simulink model "EEE4022S_Double_Pendulum_Swing_Up_SIM"  (R2021a)
settings: Solver=ode4  StartTime=0.0  StopTime=10  FixedStep=0.002  RelTol=1e-3
values from neighbouring files (symbols this model uses):
  g = 9.81    [EEE4022S_Double_Inverted_Pendulum_Model.m]    (also in MediumPenModelling.m; ShortPenModelling.m)
  K = lqr(A,B,Q,R)    [EEE4022S_Double_Inverted_Pendulum_Model.m]
  L1 = 0.2096    [EEE4022S_Double_Inverted_Pendulum_Model.m]
  l1 = 0.1483    [EEE4022S_Double_Inverted_Pendulum_Model.m]
  l2 = 0.1778    [EEE4022S_Double_Inverted_Pendulum_Model.m]
  m1 = 0.25244    [EEE4022S_Double_Inverted_Pendulum_Model.m]
  m2 = 0.10562    [EEE4022S_Double_Inverted_Pendulum_Model.m]
libraries: simulink_extras x4
settings Model: Creator=User  LastModifiedBy=User
settings SolverCC: AutoInsertRateTranBlk=on

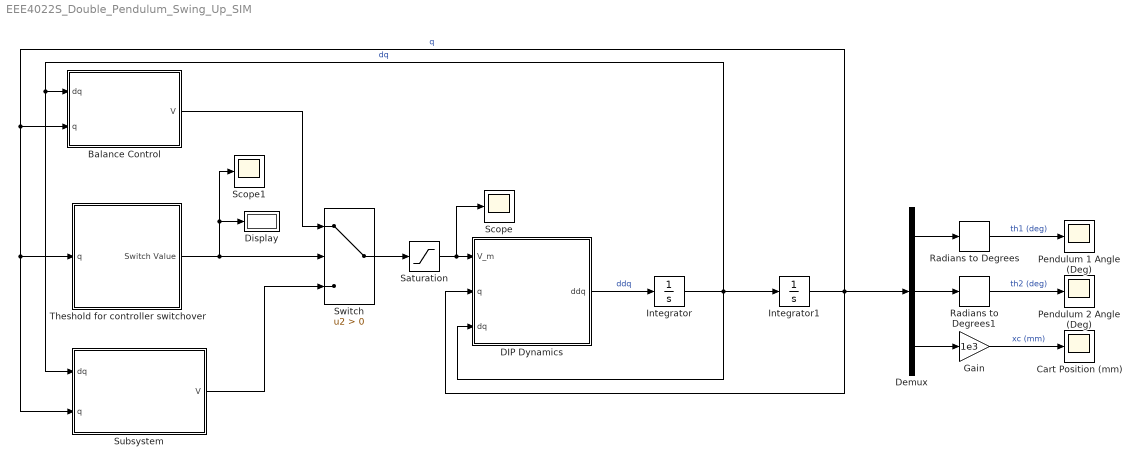
== system EEE4022S_Double_Pendulum_Swing_Up_SIM ==
  Balance Control : Subsystem
  Cart Position (mm) : Scope
  DIP Dynamics : MATLAB Function  TreatAsAtomicUnit=on
  Demux : Demux  Outputs=3
  Display : Display
  Gain : Gain  Gain=1e3
  Integrator : Integrator  InitialCondition=[0 0 0]
  Integrator1 : Integrator  InitialCondition=[5*pi/180 0*pi/180 0]
  Pendulum 1 Angle (Deg) : Scope
  Pendulum 2 Angle (Deg) : Scope
  Radians to Degrees : simulink_extras/Transformations/Radians to Degrees
  Radians to Degrees1 : simulink_extras/Transformations/Radians to Degrees
  Saturation : Saturate  UpperLimit=24  LowerLimit=-24
  Scope : Scope
  Scope1 : Scope
  Subsystem : Subsystem
  Switch : Switch  Criteria=u2 > Threshold
  Theshold for controller switchover : Subsystem
  wires:
  Demux/3 -> Gain/1
  DIP Dynamics/1(ddq) -> Integrator/1  "ddq"
  Saturation/1 -> Scope/1, DIP Dynamics/1(V_m)
  Gain/1 -> Cart Position (mm)/1  "xc (mm)"
  Integrator/1 -> DIP Dynamics/3(dq), Subsystem/1(dq), Balance Control/1(dq), Integrator1/1  "dq"
  Radians to Degrees/1 -> Pendulum 1 Angle (Deg)/1  "th1 (deg)"
  Radians to Degrees1/1 -> Pendulum 2 Angle (Deg)/1  "th2 (deg)"
  Subsystem/1(V) -> Switch/3
  Theshold for controller switchover/1(Switch Value) -> Switch/2, Scope1/1, Display/1
  Switch/1 -> Saturation/1
  Balance Control/1(V) -> Switch/1
  Demux/1 -> Radians to Degrees/1
  Demux/2 -> Radians to Degrees1/1
  Integrator1/1 -> Subsystem/2(q), Theshold for controller switchover/1(q), Balance Control/2(q), DIP Dynamics/2(q), Demux/1  "q"

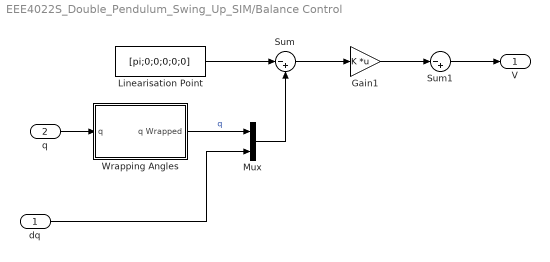
== system EEE4022S_Double_Pendulum_Swing_Up_SIM/Balance Control ==
  dq : Inport
  q : Inport  Port=2
  Gain1 : Gain  Gain=K  Multiplication=Matrix(K*u)
  Linearisation Point : Constant  Value=[pi;0;0;0;0;0]
  Mux : Mux  Inputs=2
  Sum : Sum  Inputs=|-+
  Sum1 : Sum  Inputs=|-+
  Wrapping Angles : Subsystem
  V : Outport
  wires:
  Mux/1 -> Sum/2
  dq/1 -> Mux/2
  Linearisation Point/1 -> Sum/1
  Sum/1 -> Gain1/1
  Gain1/1 -> Sum1/1
  q/1 -> Wrapping Angles/1(q)
  Sum1/1 -> V/1
  Wrapping Angles/1(q Wrapped) -> Mux/1  "q"

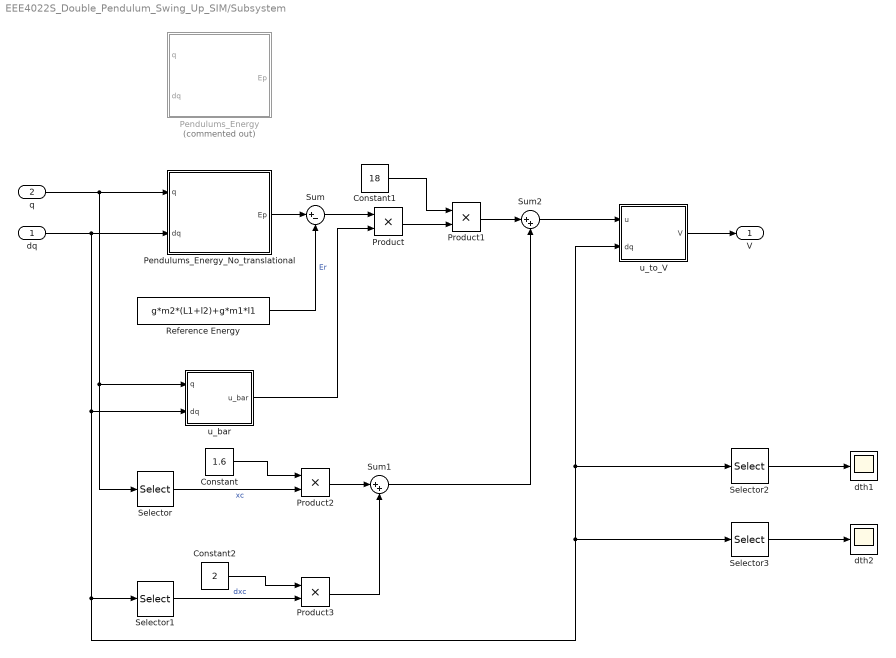
== system EEE4022S_Double_Pendulum_Swing_Up_SIM/Subsystem ==
  dq : Inport
  q : Inport  Port=2
  Constant : Constant  Value=1.6
  Constant1 : Constant  Value=18
  Constant2 : Constant  Value=2
  Pendulums_Energy : MATLAB Function  Commented=on  TreatAsAtomicUnit=on
  Pendulums_Energy_No_translational : MATLAB Function  TreatAsAtomicUnit=on
  Product{,1..3} (4 alike) : Product
  Reference Energy : Constant  Value=g*m2*(L1+l2)+g*m1*l1
  Selector : Selector  InputPortWidth=3  IndexOptions=Index vector (dialog)  Indices=[3]  OutputSizes=1
  Selector1 : Selector  InputPortWidth=3  IndexOptions=Index vector (dialog)  Indices=[3]  OutputSizes=1
  Selector2 : Selector  InputPortWidth=3  IndexOptions=Index vector (dialog)  Indices=[1]  OutputSizes=1
  Selector3 : Selector  InputPortWidth=3  IndexOptions=Index vector (dialog)  Indices=[2]  OutputSizes=1
  Sum : Sum  Inputs=|+-
  Sum1 : Sum  Inputs=|++
  Sum2 : Sum  Inputs=|++
  dth1 : Scope
  dth2 : Scope
  u_bar : MATLAB Function  TreatAsAtomicUnit=on
  u_to_V : MATLAB Function  TreatAsAtomicUnit=on
  V : Outport
  wires:
  Constant1/1 -> Product1/1
  Pendulums_Energy_No_translational/1(Ep) -> Sum/1
  Reference Energy/1 -> Sum/2  "Er"
  dq/1 -> Pendulums_Energy_No_translational/2(dq), u_bar/2(dq), Selector1/1, Selector3/1, u_to_V/2(dq), Selector2/1
  Product/1 -> Product1/2
  u_bar/1(u_bar) -> Product/2
  Sum/1 -> Product/1
  q/1 -> Pendulums_Energy_No_translational/1(q), u_bar/1(q), Selector/1
  Selector/1 -> Product2/2  "xc"
  Selector1/1 -> Product3/2  "dxc"
  Constant/1 -> Product2/1
  Constant2/1 -> Product3/1
  Product2/1 -> Sum1/1
  Product3/1 -> Sum1/2
  Product1/1 -> Sum2/1
  Sum1/1 -> Sum2/2
  Sum2/1 -> u_to_V/1(u)
  u_to_V/1(V) -> V/1
  Selector2/1 -> dth1/1
  Selector3/1 -> dth2/1

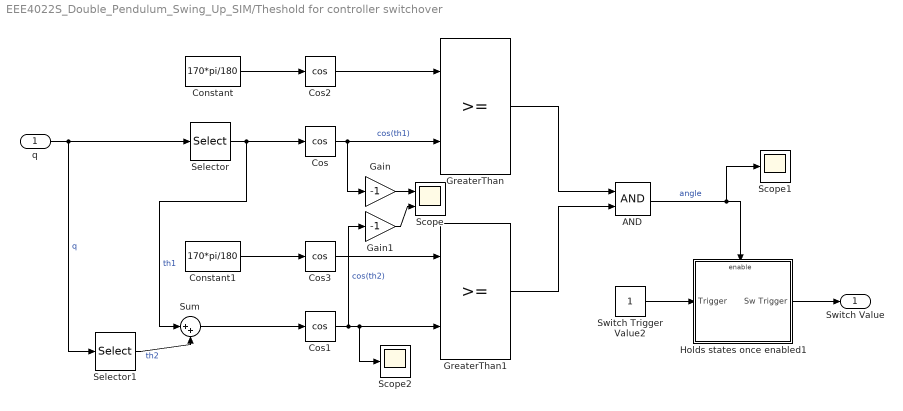
== system EEE4022S_Double_Pendulum_Swing_Up_SIM/Theshold for controller switchover ==
  q : Inport
  AND : Logic  AllPortsSameDT=off  OutDataTypeStr=boolean
  Constant : Constant  Value=170*pi/180
  Constant1 : Constant  Value=170*pi/180
  Cos{,1..3} (4 alike) : Trigonometry  Operator=cos
  Gain : Gain  Gain=-1
  Gain1 : Gain  Gain=-1
  GreaterThan : RelationalOperator  OutDataTypeStr=boolean  RndMeth=Simplest
  GreaterThan1 : RelationalOperator  OutDataTypeStr=boolean  RndMeth=Simplest
  Holds states once enabled1 : Subsystem  TreatAsAtomicUnit=on
  Scope : Scope  NumInputPorts=2
  Scope1 : Scope
  Scope2 : Scope
  Selector : Selector  InputPortWidth=3  IndexOptions=Index vector (dialog)  Indices=[1]  OutputSizes=1
  Selector1 : Selector  InputPortWidth=3  IndexOptions=Index vector (dialog)  Indices=[2]  OutputSizes=1
  Sum : Sum  Inputs=|++
  Switch Trigger Value2 : Constant
  Switch Value : Outport
  wires:
  q/1 -> Selector/1, Selector1/1  "q"
  Selector/1 -> Sum/1, Cos/1  "th1"
  Constant/1 -> Cos2/1
  Constant1/1 -> Cos3/1
  Cos2/1 -> GreaterThan/1
  Cos/1 -> GreaterThan/2, Gain/1  "cos(th1)"
  Cos1/1 -> Scope2/1, GreaterThan1/2, Gain1/1  "cos(th2)"
  Cos3/1 -> GreaterThan1/1
  GreaterThan/1 -> AND/1
  GreaterThan1/1 -> AND/2
  AND/1 -> Scope1/1, Holds states once enabled1/Enable  "angle"
  Switch Trigger Value2/1 -> Holds states once enabled1/1(Trigger)
  Holds states once enabled1/1(Sw Trigger) -> Switch Value/1
  Gain/1 -> Scope/1
  Selector1/1 -> Sum/2  "th2"
  Sum/1 -> Cos1/1
  Gain1/1 -> Scope/2

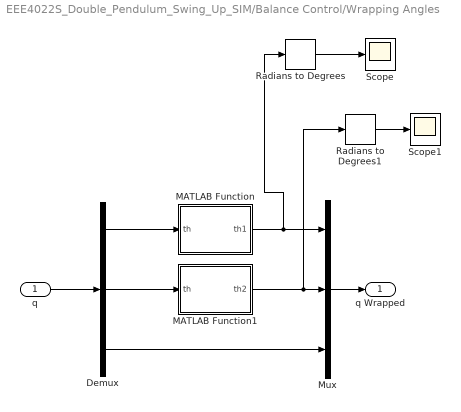
== system EEE4022S_Double_Pendulum_Swing_Up_SIM/Balance Control/Wrapping Angles ==
  q : Inport
  Demux : Demux  Outputs=3
  MATLAB Function : MATLAB Function  TreatAsAtomicUnit=on
  MATLAB Function1 : MATLAB Function  TreatAsAtomicUnit=on
  Mux : Mux  Inputs=3
  Radians to Degrees : simulink_extras/Transformations/Radians to Degrees
  Radians to Degrees1 : simulink_extras/Transformations/Radians to Degrees
  Scope : Scope
  Scope1 : Scope
  q Wrapped : Outport
  wires:
  q/1 -> Demux/1
  Mux/1 -> q Wrapped/1
  Demux/1 -> MATLAB Function/1(th)
  MATLAB Function/1(th1) -> Radians to Degrees/1, Mux/1
  Demux/2 -> MATLAB Function1/1(th)
  MATLAB Function1/1(th2) -> Radians to Degrees1/1, Mux/2
  Demux/3 -> Mux/3
  Radians to Degrees/1 -> Scope/1
  Radians to Degrees1/1 -> Scope1/1

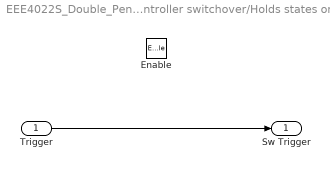
== system EEE4022S_Double_Pendulum_Swing_Up_SIM/Theshold for controller switchover/Holds states once enabled1 ==
  Trigger : Inport  OutDataTypeStr=double
  Enable : EnablePort
  Sw Trigger : Outport  OutDataTypeStr=double  InitialOutput=[0]
  wires:
  Trigger/1 -> Sw Trigger/1

== matlab function EEE4022S_Double_Pendulum_Swing_Up_SIM/Subsystem/Pendulums_Energy_No_translational ==
  data: q input; Ep output; dq input
function Ep = Pendulums_Energy_No_translational(q,dq)
%#codegen

%    This function was generated by the Symbolic Math Toolbox version 8.7.
%    31-Oct-2022 16:44:23

th1 = q(1);
th2 = q(2);
dth1 = dq(1);
dth2 = dq(2);

g = 9.81;
l1 = 0.1483;
L1 = 0.2096;
l2 = 0.1778;
m1 = 0.25244;
m2 = 0.10562;
J1 = 0.0011;
J2 = 8.2572e-04;

t2 = cos(th1);
Ep = (J1.*dth1.^2)./2.0-g.*m2.*(L1.*t2+l2.*cos(th1+th2))+J2.*(dth1+dth2).*(dth1./2.0+dth2./2.0)-g.*l1.*m1.*t2;

== matlab function EEE4022S_Double_Pendulum_Swing_Up_SIM/Subsystem/Pendulums_Energy ==
  data: q input; Ep output; dq input
function Ep = Pendulums_Energy(q,dq)
%#codegen

%    This function was generated by the Symbolic Math Toolbox version 8.7.
%    31-Oct-2022 14:17:52

th1 = q(1);
th2 = q(2);
dth1 = dq(1);
dth2 = dq(2);

g = 9.81;
l1 = 0.1483;
L1 = 0.2096;
l2 = 0.1778;
m1 = 0.25244;
m2 = 0.10562;
J1 = 0.0011;
J2 = 8.2572e-04;

t2 = cos(th1);
t3 = cos(th2);
t4 = dth1.^2;
t5 = dth2.^2;
t6 = l2.^2;
Ep = (J1.*t4)./2.0+(J2.*t4)./2.0+(J2.*t5)./2.0+(l1.^2.*m1.*t4)./2.0+J2.*dth1.*dth2+(m2.*t4.*t6)./2.0+(m2.*t5.*t6)./2.0+(L1.^2.*m2.*t4)./2.0+dth1.*dth2.*m2.*t6-g.*l1.*m1.*t2-L1.*g.*m2.*t2+L1.*l2.*m2.*t3.*t4+g.*l2.*m2.*sin(th1).*sin(th2)-g.*l2.*m2.*t2.*t3+L1.*dth1.*dth2.*l2.*m2.*t3;

== matlab function EEE4022S_Double_Pendulum_Swing_Up_SIM/Subsystem/u_bar ==
  data: q input; u_bar output; dq input
function u_bar = u_bar(q,dq)
%#codegen

%    This function was generated by the Symbolic Math Toolbox version 8.7.
%    31-Oct-2022 18:22:34

th1 = q(1);
th2 = q(2);
dth1 = dq(1);
dth2 = dq(2);

l1 = 0.1483;
L1 = 0.2096;
l2 = 0.1778;
m1 = 0.25244;
m2 = 0.10562;

t2 = cos(th1);
t3 = th1+th2;
t4 = cos(t3);
u_bar = dth1.*l1.*m1.*t2+dth1.*l2.*m2.*t4+dth2.*l2.*m2.*t4+L1.*dth1.*m2.*t2;

== matlab function EEE4022S_Double_Pendulum_Swing_Up_SIM/Subsystem/u_to_V ==
  data: u input; dq input; V output
function V = u_to_V(u,dq)
%#codegen

%    This function was generated by the Symbolic Math Toolbox version 8.7.
%    31-Oct-2022 18:30:42

dx = dq(3);
mc = 0.57;

R_m = 2.6; 
k_t = 0.00767;
n_m = 1;
k_m = 0.00767;
K_g = 3.71;
n_g = 1;
r_mp = 6.35*10^(-3);

V = (K_g.*dx.*k_m)./r_mp+(R_m.*mc.*r_mp.*u)./(K_g.*k_t.*n_g.*n_m);

== matlab function EEE4022S_Double_Pendulum_Swing_Up_SIM/Balance Control/Wrapping Angles/MATLAB Function ==
  data: th input; th1 output
function th1 = wrapth(th)

th1 = wrapTo2Pi(th);

== matlab function EEE4022S_Double_Pendulum_Swing_Up_SIM/Balance Control/Wrapping Angles/MATLAB Function1 ==
  data: th input; th2 output
function th2 = wrapth(th)

th2 = wrapToPi(th);

== matlab function EEE4022S_Double_Pendulum_Swing_Up_SIM/DIP Dynamics ==
  data: V_m input; ddq output; q input; dq input
function ddq = Dynamics(V_m,q,dq)
%#codegen

%    This function was generated by the Symbolic Math Toolbox version 8.7.
%    26-Sep-2022 15:32:26

Bc = 9.3378;
Bp1 = 5.6134e-04;
Bp2 = 4.2362e-04;
Cp1 = 0;
Cp2 = 0;
J1 = 0.0011;
J2 = 8.25272e-04;

sgn1 = 0;
sgn2 = 0;

th1 = q(1);
th2 = q(2);

dth1 = dq(1);
dth2 = dq(2);
dx = dq(3);

if dth1 > 0
    sgn1 = 1;
elseif dth1 == 0
    sgn1 = 0;
elseif dth1 < 0
    sgn1 = -1;
end

if dth2 > 0
    sgn2 = 1;
elseif dth2 == 0
    sgn2 = 0;
elseif dth2 < 0
    sgn2 = -1;
end

t2 = cos(th1);
t3 = cos(th2);
t4 = sin(th1);
t5 = sin(th2);
t6 = th1+th2;
t7 = dth1.^2;
t8 = dth2.^2;
t9 = th1.*2.0;
t10 = th2.*2.0;
t17 = -th2;
t31 = J2.*2.40131524463645e+27;
t33 = J1.*9.132544930438125e+26;
t36 = J1.*J2.*2.9001875e+29;
t11 = cos(t9);
t12 = cos(t10);
t13 = sin(t9);
t14 = sin(t10);
t15 = cos(t6);
t16 = sin(t6);
t18 = t6+th2;
t19 = t6+th1;
t24 = t17+th1;
t25 = t6.*2.0;
t20 = cos(t18);
t21 = cos(t19);
t22 = sin(t18);
t23 = sin(t19);
t26 = cos(t24);
t27 = sin(t24);
t28 = cos(t25);
t29 = sin(t25);
t30 = t12.*1.558579647284476e+24;
t32 = t11.*1.163567673749033e+24;
t37 = J2.*t11.*5.545558236935025e+26;
t34 = -t30;
t35 = -t32;
t38 = t28.*1.264549000462369e+23;
t39 = -t37;
t40 = J1.*t28.*5.51030788662025e+25;
t41 = -t40;
t42 = t31+t33+t34+t35+t36+t38+t39+t41+5.897676898508321e+24;
t43 = 1.0./t42;
et1 = J1.*4.566272465219062e+26+J2.*1.200657622318225e+27-t11.*5.817838368745163e+23-t12.*7.792898236422378e+23+t28.*6.322745002311845e+22-J2.*t11.*2.772779118467512e+26;
et2 = J1.*t28.*-2.755153943310125e+25+J1.*J2.*1.45009375e+29+2.948838449254161e+24;
et3 = t4.*1.72814792752668e+30-t22.*2.941400624947678e+29+Bp1.*dth1.*3.682470429575913e+30-Bp2.*dth2.*3.682470429575913e+30+J2.*t4.*6.834474957640116e+32;
et4 = V_m.*t2.*3.517412247307424e+29-V_m.*t20.*8.026695626668189e+28+Cp1.*sgn1.*3.682470429575913e+30-Cp2.*sgn2.*3.682470429575913e+30-dx.*t2.*1.576227207648911e+30;
et5 = dx.*t20.*3.596932956594992e+29-t5.*t7.*1.214115554643148e+28-t5.*t8.*1.214115554643148e+28+t7.*t13.*4.691795752474537e+27-t7.*t14.*6.284582782762827e+27;
et6 = t7.*t23.*1.478953077202183e+27+t8.*t23.*1.478953077202183e+27+Bp1.*J2.*dth1.*1.1694281046875e+33-Bp2.*J2.*dth2.*1.1694281046875e+33+J2.*V_m.*t2.*1.293845127843844e+32;
et7 = Bc.*dx.*t2.*-2.040802939412686e+29+Bc.*dx.*t20.*4.657089609332816e+28-Bp2.*dth2.*t3.*3.898150186249388e+30+Bp2.*dth2.*t21.*7.04868363426875e+29-Bp1.*dth1.*t28.*2.22189389758245e+29;
et8 = Bp2.*dth2.*t28.*2.22189389758245e+29+J2.*Cp1.*sgn1.*1.1694281046875e+33-J2.*Cp2.*sgn2.*1.1694281046875e+33-J2.*dx.*t2.*5.797995087304892e+32-J2.*t5.*t7.*3.898150186249388e+30;
et9 = J2.*t5.*t8.*-3.898150186249388e+30+J2.*t7.*t13.*2.236107720088125e+30+J2.*t7.*t23.*7.04868363426875e+29+J2.*t8.*t23.*7.04868363426875e+29-dth1.*dth2.*t5.*2.428231109286297e+28;
et10 = dth1.*dth2.*t23.*2.957906154404366e+27-Cp2.*sgn2.*t3.*3.898150186249388e+30+Cp2.*sgn2.*t21.*7.04868363426875e+29-Cp1.*sgn1.*t28.*2.22189389758245e+29+Cp2.*sgn2.*t28.*2.22189389758245e+29;
et11 = Bc.*J2.*dx.*t2.*-7.50689073215625e+31-J2.*dth1.*dth2.*t5.*7.796300372498775e+30+J2.*dth1.*dth2.*t23.*1.40973672685375e+30;
et12 = t4.*-3.456295855053359e+30+t16.*8.774418773455151e+29+t22.*5.882801249895356e+29-t27.*1.866245950758971e+30-Bp1.*dth1.*7.364940859151826e+30;
et13 = Bp2.*dth2.*2.673034764952248e+31-J2.*t4.*1.366894991528023e+33+J1.*t16.*4.308741600412609e+32-V_m.*t2.*7.034824494614848e+29+V_m.*t15.*3.220819427635901e+29;
et14 = V_m.*t20.*1.605339125333638e+29-V_m.*t26.*5.092739861476948e+29-Cp1.*sgn1.*7.364940859151826e+30+Cp2.*sgn2.*2.673034764952248e+31+dx.*t2.*3.152454415297823e+30;
et15 = dx.*t15.*-1.443317659637463e+30-dx.*t20.*7.193865913189984e+29+dx.*t26.*2.282165002775269e+30+t5.*t7.*8.613899182297017e+28+t5.*t8.*2.428231109286297e+28;
et16 = t7.*t13.*-9.383591504949074e+27+t7.*t14.*2.513833113105131e+28+t8.*t14.*1.256916556552565e+28-t7.*t23.*6.193081403298507e+27-t8.*t23.*2.957906154404366e+27-t7.*t29.*1.019795541422878e+27;
et17 = t8.*t29.*(-1.019795541422878e+27)-Bp1.*J2.*dth1.*2.338856209375e+33+Bp2.*J1.*dth2.*2.338856209375e+33+Bp2.*J2.*dth2.*2.338856209375e+33-J2.*V_m.*t2.*2.587690255687688e+32;
et18 = J1.*V_m.*t15.*8.156946014704375e+31+Bc.*dx.*t2.*4.081605878825372e+29-Bc.*dx.*t15.*1.868719755629583e+29-Bc.*dx.*t20.*9.314179218665632e+28+Bc.*dx.*t26.*2.95480817948546e+29;
et19 = Bp1.*dth1.*t3.*-7.796300372498775e+30+Bp2.*dth2.*t3.*1.559260074499755e+31-Bp2.*dth2.*t11.*4.472215440176251e+30+Bp1.*dth1.*t21.*1.40973672685375e+30-Bp2.*dth2.*t21.*2.8194734537075e+30;
et20 = Bp1.*dth1.*t28.*4.443787795164901e+29-Bp2.*dth2.*t28.*4.443787795164901e+29-J2.*Cp1.*sgn1.*2.338856209375e+33+J1.*Cp2.*sgn2.*2.338856209375e+33+J2.*Cp2.*sgn2.*2.338856209375e+33;
et21 = J2.*dx.*t2.*1.159599017460978e+33-J1.*dx.*t15.*3.655300924576745e+32+J1.*t5.*t7.*7.796300372498775e+30+J2.*t5.*t7.*7.796300372498775e+30+J2.*t5.*t8.*7.796300372498775e+30;
et22 = J2.*t7.*t13.*-4.472215440176251e+30+J1.*t7.*t23.*1.40973672685375e+30-J2.*t7.*t23.*1.40973672685375e+30-J2.*t8.*t23.*1.40973672685375e+30+J1.*t7.*t29.*4.443787795164901e+29;
et23 = J1.*t8.*t29.*4.443787795164901e+29+dth1.*dth2.*t5.*4.856462218572593e+28+dth1.*dth2.*t14.*2.513833113105131e+28-dth1.*dth2.*t23.*5.915812308808732e+27-dth1.*dth2.*t29.*2.039591082845755e+27;
et24 = Cp1.*sgn1.*t3.*-7.796300372498775e+30+Cp2.*sgn2.*t3.*1.559260074499755e+31-Cp2.*sgn2.*t11.*4.472215440176251e+30+Cp1.*sgn1.*t21.*1.40973672685375e+30-Cp2.*sgn2.*t21.*2.8194734537075e+30;
et25 = Cp1.*sgn1.*t28.*4.443787795164901e+29-Cp2.*sgn2.*t28.*4.443787795164901e+29+Bc.*J2.*dx.*t2.*1.50137814643125e+32-Bc.*J1.*dx.*t15.*4.7326608975625e+31+J2.*dth1.*dth2.*t5.*1.559260074499755e+31;
et26 = J2.*dth1.*dth2.*t23.*-2.8194734537075e+30+J1.*dth1.*dth2.*t29.*8.887575590329801e+29;
et27 = V_m.*5.70835880467167e+32-dx.*2.558036939182608e+33+t13.*4.602651633177521e+32-t29.*5.002097130679214e+31-Bc.*dx.*3.311990352201115e+32;
et28 = J1.*dx.*-3.249562521948726e+35-J2.*dx.*9.919153959225849e+35+J2.*t13.*2.193621673406451e+35+J1.*t29.*2.179677913528384e+34-V_m.*t12.*1.682395403349653e+32;
et29 = dx.*t12.*7.539171477023103e+32+t4.*t7.*1.498461192925065e+31+t7.*t16.*1.286689177165899e+30+t8.*t16.*1.286689177165899e+30-t7.*t22.*1.068745727411176e+30;
et30 = t7.*t27.*3.099885649815775e+30+t8.*t27.*3.099885649815775e+30+J1.*V_m.*7.251525007072189e+34+J2.*V_m.*2.213497740033953e+35+J1.*J2.*V_m.*2.17179921875e+37;
et31 = Bc.*J1.*dx.*-4.207335537933063e+34-Bc.*J2.*dx.*1.284271611239947e+35-J1.*J2.*dx.*9.7322940203125e+37+Bc.*dx.*t12.*9.761259821161582e+31+Bp1.*dth1.*t2.*2.040802939412686e+33;
et32 = Bp2.*dth2.*t2.*-2.040802939412686e+33+Bp2.*dth2.*t15.*9.343598778147914e+32-Bp1.*dth1.*t20.*4.657089609332816e+32+Bp2.*dth2.*t20.*4.657089609332816e+32-Bp2.*dth2.*t26.*1.47740408974273e+33;
et33 = J1.*t4.*t7.*2.040802939412686e+33+J2.*t4.*t7.*7.651022952238403e+33+J1.*t7.*t16.*7.901054699803193e+32+J1.*t8.*t16.*7.901054699803193e+32+J2.*t7.*t16.*9.343598778147914e+32;
et34 = J2.*t8.*t16.*9.343598778147914e+32+J1.*t7.*t22.*4.657089609332816e+32+J2.*t7.*t27.*1.47740408974273e+33+J2.*t8.*t27.*1.47740408974273e+33+dth1.*dth2.*t16.*2.573378354331798e+30;
et35 = dth1.*dth2.*t27.*6.199771299631551e+30+Cp1.*sgn1.*t2.*2.040802939412686e+33-Cp2.*sgn2.*t2.*2.040802939412686e+33+Cp2.*sgn2.*t15.*9.343598778147914e+32-Cp1.*sgn1.*t20.*4.657089609332816e+32;
et36 = Cp2.*sgn2.*t20.*4.657089609332816e+32-Cp2.*sgn2.*t26.*1.47740408974273e+33-Bc.*J1.*J2.*dx.*1.260078125e+37+Bp1.*J2.*dth1.*t2.*7.50689073215625e+35;
et37 = Bp2.*J2.*dth2.*t2.*-7.50689073215625e+35+Bp2.*J1.*dth2.*t15.*2.36633044878125e+35+J1.*J2.*t4.*t7.*7.50689073215625e+35+J1.*J2.*t7.*t16.*2.36633044878125e+35;
et38 = J1.*J2.*t8.*t16.*2.36633044878125e+35+J1.*dth1.*dth2.*t16.*1.580210939960639e+33+J2.*dth1.*dth2.*t16.*1.868719755629583e+33+J2.*dth1.*dth2.*t27.*2.95480817948546e+33+J2.*Cp1.*sgn1.*t2.*7.50689073215625e+35;
et39 = J2.*Cp2.*sgn2.*t2.*-7.50689073215625e+35+J1.*Cp2.*sgn2.*t15.*2.36633044878125e+35+J1.*J2.*dth1.*dth2.*t16.*4.7326608975625e+35;
ddq = [((et3+et4+et5+et6+et7+et8+et9+et10+et11).*(-1.24000248000496e-4))./(et1+et2);t43.*(et12+et13+et14+et15+et16+et17+et18+et19+et20+et21+et22+et23+et24+et25+et26).*(-1.24000248000496e-4);(t43.*(et27+et28+et29+et30+et31+et32+et33+et34+et35+et36+et37+et38+et39))./4.03225e+7];
